simulink model "Model_IPS"  (Simulink 7.8)
settings: Solver=ode45  StartTime=0.0  StopTime=4  MaxStep=0.00001  RelTol=1e-3
values from neighbouring files (symbols this model uses):
  Imrn = 7.4    [parametriAM.m]
  Ismax = In*sqrt(2)    [parametriAM.m]
  J = 0.019    [parametriAM.m]
  Lm = 0.0493    [parametriAM.m]
  Lr = 0.05315    [parametriAM.m]
  Ls = 0.05315    [parametriAM.m]
  Ls_oc = Ls    (= 0.05315)    [parametriAM.m]
  pp = 3    [parametriAM.m]
  Rs = 0.594    [parametriAM.m]
  Rs_oc = Rs    (= 0.594)    [parametriAM.m]
  sigma = 1 - 1/((1+sigmaR)*(1+sigmaS))    (= 0.13962595434)    [parametriAM.m]
  sigma_oc = 1 - 1/((1+sigmaR_oc)*(1+sigmaS_oc))    (= 0.13962595434)    [parametriAM.m]
  Tr = Lr/Rr    (= 0.0771407837446)    [parametriAM.m]
  Usmax = Udc    [parametriAM.m]
libraries: simulink x5
settings Model: Creator=Vaje  LastModifiedBy=Mitja1  CovModelRefEnable=off
settings DataIOCC: LimitDataPoints=off  SaveFormat=StructureWithTime  SignalLoggingSaveFormat=Dataset
settings OptimizationCC: ExpressionDepthLimit=128
settings DebuggingCC: UnderspecifiedInitializationDetection=Simplified  MergeDetectMultiDrivingBlocksExec=error  SolverPrmCheckMsg=none  FrameProcessingCompatibilityMsg=error  StateNameClashWarn=none
settings HardwareCC: ProdBitPerPointer=64  ProdLargestAtomicFloat=Float  ProdIntDivRoundTo=Zero  ProdEndianess=LittleEndian  ProdHWDeviceType=Specified
settings CodeAppCC: CustomSymbolStrType=$N$R$M_T
settings GRTTargetCC: TargetFunctionLibrary=C89/C90 (ANSI)

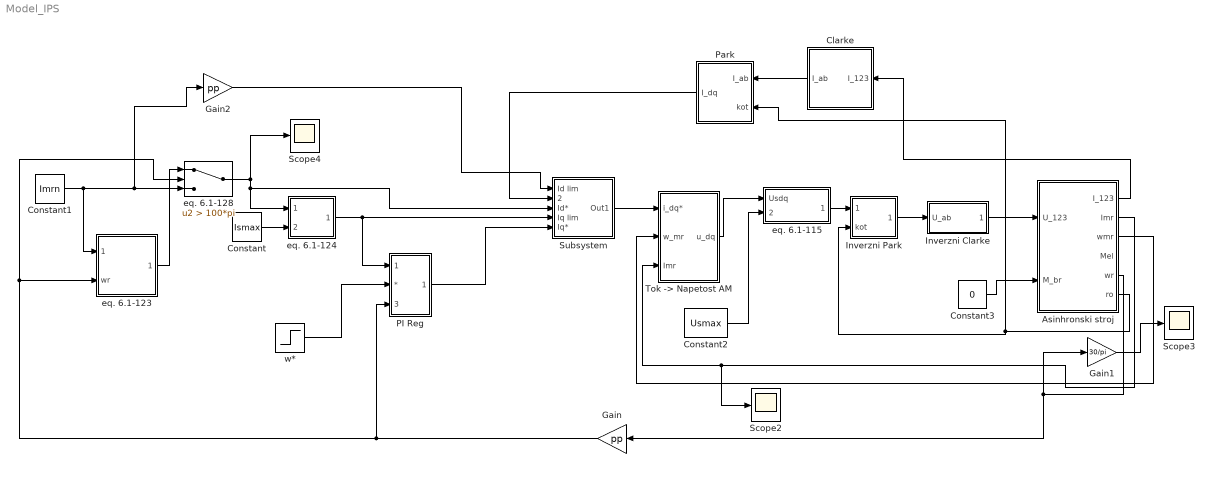
== system Model_IPS ==
  Asinhronski stroj : Subsystem  InitFcn=parametriAM
  Clarke : Subsystem
  Constant : Constant  Value=Ismax
  Constant1 : Constant  Value=Imrn
  Constant2 : Constant  Value=Usmax
  Constant3 : Constant  Value=0
  Gain : Gain  Gain=pp
  Gain1 : Gain  Gain=30/pi
  Gain2 : Gain  Gain=pp
  Inverzni Clarke : Subsystem
  Inverzni Park : Subsystem
  PI Reg : Subsystem
  Park : Subsystem
  Scope2 : Scope
      settings: TimeRange=auto  MaxDataPoints=5000  SaveToWorkspace=off  SaveName=ScopeData2  YMin=8.68295  YMax=8.68443  SampleTime=-1
  Scope3 : Scope
      settings: TimeRange=auto  MaxDataPoints=5000  SaveToWorkspace=off  SaveName=ScopeData3  YMin=-1.00000  YMax=1.00000  SampleTime=-1
  Scope4 : Scope
      settings: TimeRange=auto  MaxDataPoints=5000  SaveToWorkspace=off  SaveName=ScopeData2  YMin=0  YMax=10  SampleTime=-1
  Subsystem : Subsystem
  "Tok -> Napetost AM" : Subsystem
  eq. 6.1-115 : Subsystem
  eq. 6.1-123 : Subsystem
  eq. 6.1-124 : Subsystem
  eq. 6.1-128 : Switch  Criteria=u2 > Threshold  Threshold=100*pi
  w* : Step  Time=0.3  After=200*pi  SampleTime=0
  wires:
  Inverzni Clarke/1(U_123) -> Asinhronski stroj/1(U_123)
  Asinhronski stroj/1(I_123) -> Clarke/1(I_123)
  Asinhronski stroj/6(ro) -> Park/2(kot), Inverzni Park/2(kot)
  Inverzni Park/1(U_ab) -> Inverzni Clarke/1(U_ab)
  eq. 6.1-115/1(Usdqlim) -> Inverzni Park/1(U_dq)
  eq. 6.1-128/1 -> Subsystem/3(Id*), eq. 6.1-124/1(Isdref), Scope4/1
  eq. 6.1-123/1(Isdref) -> eq. 6.1-128/1
  Constant/1 -> eq. 6.1-124/2(Ismax)
  Constant1/1 -> eq. 6.1-123/1(Isdrated), Gain2/1, eq. 6.1-128/3
  Gain/1 -> eq. 6.1-128/2, eq. 6.1-123/2(wr), PI Reg/3(dej)
  Constant2/1 -> eq. 6.1-115/2(Usmax)
  Asinhronski stroj/5(wr) -> Gain1/1, Gain/1
  eq. 6.1-124/1(Isq lim) -> PI Reg/1(Sat), Subsystem/4(Iq lim)
  Clarke/1(I_ab) -> Park/1(I_ab)
  "Tok -> Napetost AM"/1(u_dq) -> eq. 6.1-115/1(Usdq)
  Asinhronski stroj/2(Imr) -> Scope2/1, "Tok -> Napetost AM"/3(Imr)
  Asinhronski stroj/3(wmr) -> "Tok -> Napetost AM"/2(w_mr)
  Gain1/1 -> Scope3/1
  Constant3/1 -> Asinhronski stroj/2(M_br)
  w*/1 -> PI Reg/2(*)
  Gain2/1 -> Subsystem/1(Id lim)
  Park/1(I_dq) -> Subsystem/2(Idq dej)
  PI Reg/1(Out) -> Subsystem/5(Iq*)
  Subsystem/1(Out1) -> "Tok -> Napetost AM"/1(i_dq*)

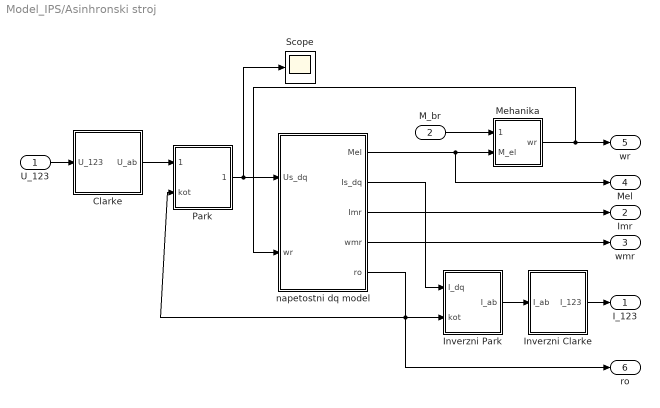
== system Model_IPS/Asinhronski stroj ==
  U_123 : Inport
  M_br : Inport  Port=2
  Clarke : Subsystem
  Inverzni Clarke : Subsystem
  Inverzni Park : Subsystem
  Mehanika : Subsystem
  Park : Subsystem
  Scope : Scope
      settings: TimeRange=auto  MaxDataPoints=5000  SaveToWorkspace=off  SaveName=ScopeData  YMin=-1.00000  YMax=1.00000  SampleTime=-1
  napetostni dq model : Subsystem
  I_123 : Outport
  Imr : Outport  Port=2
  wmr : Outport  Port=3
  Mel : Outport  Port=4
  wr : Outport  Port=5
  ro : Outport  Port=6
  wires:
  Inverzni Park/1(I_ab) -> Inverzni Clarke/1(I_ab)
  Clarke/1(U_ab) -> Park/1(U_ab)
  Mehanika/1(wr) -> napetostni dq model/2(wr), wr/1
  M_br/1 -> Mehanika/1(M_br)
  napetostni dq model/1(Mel) -> Mel/1, Mehanika/2(M_el)
  Inverzni Clarke/1(I_123) -> I_123/1
  napetostni dq model/4(wmr) -> wmr/1
  napetostni dq model/3(Imr) -> Imr/1
  U_123/1 -> Clarke/1(U_123)
  napetostni dq model/2(Is_dq) -> Inverzni Park/1(I_dq)
  napetostni dq model/5(ro) -> ro/1, Park/2(kot), Inverzni Park/2(kot)
  Park/1(U_dq) -> Scope/1, napetostni dq model/1(Us_dq)

== system Model_IPS/Clarke ==
  I_123 : Inport
  ABC_ab1 : Subsystem
  Demux : Demux  Outputs=3
  Mux : Mux  Inputs=2
  I_ab : Outport
  wires:
  Mux/1 -> I_ab/1
  ABC_ab1/2(beta) -> Mux/2
  ABC_ab1/1(alfa) -> Mux/1
  Demux/3 -> ABC_ab1/3(C)
  Demux/2 -> ABC_ab1/2(B)
  Demux/1 -> ABC_ab1/1(A)
  I_123/1 -> Demux/1

== system Model_IPS/Inverzni Clarke ==
  U_ab : Inport
  Demux : Demux  Outputs=2
  Mux : Mux  Inputs=3
  ab_ABC : Subsystem
  U_123 : Outport
  wires:
  ab_ABC/3(C) -> Mux/3
  ab_ABC/2(B) -> Mux/2
  ab_ABC/1(A) -> Mux/1
  Demux/2 -> ab_ABC/2(beta)
  Demux/1 -> ab_ABC/1(alfa)
  U_ab/1 -> Demux/1
  Mux/1 -> U_123/1

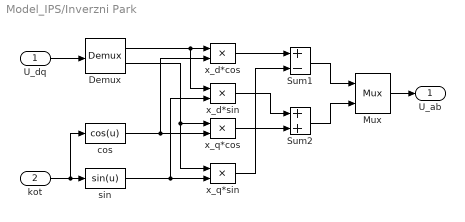
== system Model_IPS/Inverzni Park ==
  U_dq : Inport
  kot : Inport  Port=2
  Demux : Demux  Outputs=2
  Mux : Mux  Inputs=2
  "Sum1 " : Sum  Inputs=+-  SaturateOnIntegerOverflow=on  InputSameDT=on  OutDataTypeStr=Inherit: Same as first input
  Sum2 : Sum  SaturateOnIntegerOverflow=on  InputSameDT=on  OutDataTypeStr=Inherit: Same as first input
  cos : Fcn  Expr=cos(u)
  sin : Fcn  Expr=sin(u)
  x_d*cos : Product  SaturateOnIntegerOverflow=on  RndMeth=Zero  InputSameDT=on  OutDataTypeStr=Inherit: Same as first input
  x_d*sin : Product  SaturateOnIntegerOverflow=on  RndMeth=Zero  InputSameDT=on  OutDataTypeStr=Inherit: Same as first input
  x_q*cos : Product  SaturateOnIntegerOverflow=on  RndMeth=Zero  InputSameDT=on  OutDataTypeStr=Inherit: Same as first input
  "x_q*sin " : Product  SaturateOnIntegerOverflow=on  RndMeth=Zero  InputSameDT=on  OutDataTypeStr=Inherit: Same as first input
  U_ab : Outport
  wires:
  Mux/1 -> U_ab/1
  U_dq/1 -> Demux/1
  Demux/1 -> x_d*sin/1, x_d*cos/1
  Demux/2 -> "x_q*sin "/1, x_q*cos/1
  cos/1 -> x_q*cos/2, x_d*cos/2
  sin/1 -> "x_q*sin "/2, x_d*sin/2
  x_d*cos/1 -> "Sum1 "/1
  "x_q*sin "/1 -> "Sum1 "/2
  x_q*cos/1 -> Sum2/2
  x_d*sin/1 -> Sum2/1
  "Sum1 "/1 -> Mux/1
  Sum2/1 -> Mux/2
  kot/1 -> cos/1, sin/1

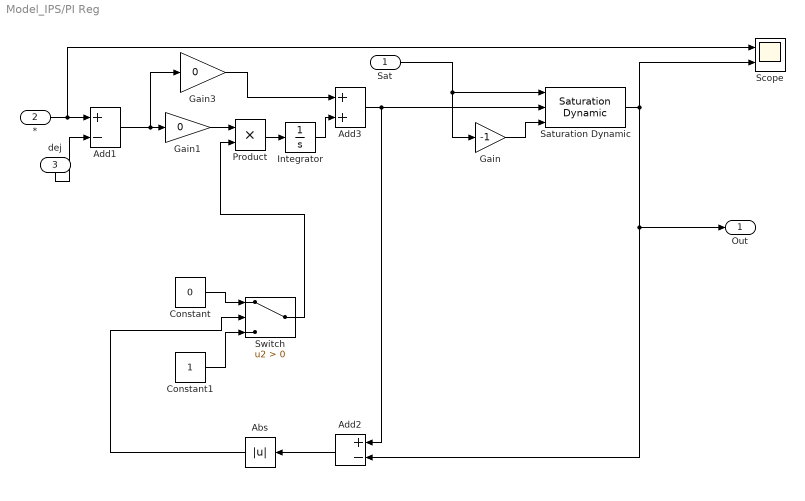
== system Model_IPS/PI Reg ==
  Sat : Inport
  * : Inport  Port=2
  dej : Inport  Port=3
  Abs : Abs
  Add1 : Sum  Inputs=+-
  Add2 : Sum  Inputs=+-
  Add3 : Sum
  Constant : Constant  Value=0
  Constant1 : Constant
  Gain : Gain  Gain=-1
  Gain1 : Gain  Gain=0
  Gain3 : Gain  Gain=0
  Integrator : Integrator
  Product : Product
  Saturation Dynamic : simulink/Discontinuities/Saturation Dynamic  OutMin=[]  OutMax=[]  OutDataTypeStr=Inherit: Same as second input  OutDataType=fixdt(1, 16)  OutScaling=2^-10  DoSatur=off
  Scope : Scope  NumInputPorts=2
      settings: TimeRange=auto  MaxDataPoints=5000  SaveToWorkspace=off  SaveName=ScopeData7  YMin=-2.0166~-5  YMax=2.47044~5  SampleTime=-1
  Switch : Switch  Criteria=u2 > Threshold  ZeroCross=off
  Out : Outport
  wires:
  Product/1 -> Integrator/1
  dej/1 -> Add1/2
  Constant1/1 -> Switch/3
  Gain3/1 -> Add3/1
  */1 -> Scope/1, Add1/1
  Saturation Dynamic/1 -> Add2/2, Out/1, Scope/2
  Add2/1 -> Abs/1
  Integrator/1 -> Add3/2
  Gain1/1 -> Product/1
  Add1/1 -> Gain1/1, Gain3/1
  Add3/1 -> Add2/1, Saturation Dynamic/2
  Switch/1 -> Product/2
  Constant/1 -> Switch/1
  Abs/1 -> Switch/2
  Sat/1 -> Saturation Dynamic/1, Gain/1
  Gain/1 -> Saturation Dynamic/3

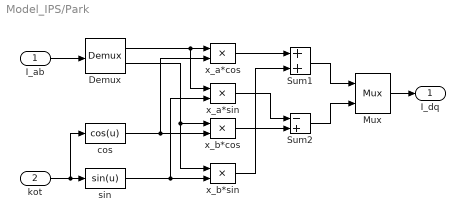
== system Model_IPS/Park ==
  I_ab : Inport
  kot : Inport  Port=2
  Demux : Demux  Outputs=2
  Mux : Mux  Inputs=2
  "Sum1 " : Sum  SaturateOnIntegerOverflow=on  InputSameDT=on  OutDataTypeStr=Inherit: Same as first input
  Sum2 : Sum  Inputs=-+  SaturateOnIntegerOverflow=on  InputSameDT=on  OutDataTypeStr=Inherit: Same as first input
  cos : Fcn  Expr=cos(u)
  sin : Fcn  Expr=sin(u)
  x_a*cos : Product  SaturateOnIntegerOverflow=on  RndMeth=Zero  InputSameDT=on  OutDataTypeStr=Inherit: Same as first input
  x_a*sin : Product  SaturateOnIntegerOverflow=on  RndMeth=Zero  InputSameDT=on  OutDataTypeStr=Inherit: Same as first input
  x_b*cos : Product  SaturateOnIntegerOverflow=on  RndMeth=Zero  InputSameDT=on  OutDataTypeStr=Inherit: Same as first input
  "x_b*sin " : Product  SaturateOnIntegerOverflow=on  RndMeth=Zero  InputSameDT=on  OutDataTypeStr=Inherit: Same as first input
  I_dq : Outport
  wires:
  Mux/1 -> I_dq/1
  I_ab/1 -> Demux/1
  Demux/1 -> x_a*sin/1, x_a*cos/1
  Demux/2 -> "x_b*sin "/1, x_b*cos/1
  cos/1 -> x_b*cos/2, x_a*cos/2
  sin/1 -> "x_b*sin "/2, x_a*sin/2
  x_a*cos/1 -> "Sum1 "/1
  "x_b*sin "/1 -> "Sum1 "/2
  x_b*cos/1 -> Sum2/2
  x_a*sin/1 -> Sum2/1
  "Sum1 "/1 -> Mux/1
  Sum2/1 -> Mux/2
  kot/1 -> cos/1, sin/1

== system Model_IPS/Subsystem ==
  Id lim : Inport
  Idq dej : Inport  Port=2
  Id* : Inport  Port=3
  Iq lim : Inport  Port=4
  Iq* : Inport  Port=5
  Demux : Demux  Outputs=2
  Mux : Mux  Inputs=2
  PI Id : Subsystem
  PI Iq : Subsystem
  Scope6 : Scope  NumInputPorts=2
      settings: TimeRange=auto  MaxDataPoints=5000  SaveToWorkspace=off  SaveName=ScopeData4  YMin=-6.22165~-5  YMax=55.99486~5  SampleTime=-1
  Out1 : Outport
  wires:
  Id*/1 -> Scope6/1, PI Id/2(*)
  Iq lim/1 -> PI Iq/1(Sat)
  PI Id/1(Out) -> Mux/1, Scope6/2
  Demux/2 -> PI Iq/3(dej)
  Iq*/1 -> PI Iq/2(*)
  Id lim/1 -> PI Id/1(Sat)
  Demux/1 -> PI Id/3(dej)
  PI Iq/1(Out) -> Mux/2
  Mux/1 -> Out1/1
  Idq dej/1 -> Demux/1

== system Model_IPS/Tok -> Napetost AM ==
  i_dq* : Inport
  w_mr : Inport  Port=2
  Imr : Inport  Port=3
  Mux : Mux  Inputs=2
  eq 5.146 : Subsystem
  eq 5.147 : Subsystem
  u_dq : Outport
  wires:
  i_dq*/1 -> eq 5.147/1(I_dq), eq 5.146/1(I_dq)
  Mux/1 -> u_dq/1
  w_mr/1 -> eq 5.147/2(w_mr), eq 5.146/2(w_mr)
  Imr/1 -> eq 5.146/3(Imr), eq 5.147/3(Imr)
  eq 5.147/1(u_q) -> Mux/2
  eq 5.146/1(u_d) -> Mux/1

== system Model_IPS/eq. 6.1-115 ==
  Usdq : Inport
  Usmax : Inport  Port=2
  Demux : Demux  Outputs=2
  Mux1 : Mux  Inputs=2
  eq. 6.1-120 : Subsystem
  eq. 6.1-120a : Subsystem
  Usdqlim : Outport
  wires:
  Mux1/1 -> Usdqlim/1
  eq. 6.1-120a/1(Usqlim) -> Mux1/2
  eq. 6.1-120/1(Usdlim) -> Mux1/1
  Usdq/1 -> Demux/1
  Demux/1 -> eq. 6.1-120a/1(Usd), eq. 6.1-120/2(Usd)
  Demux/2 -> eq. 6.1-120a/2(Usq), eq. 6.1-120/1(Usq)
  Usmax/1 -> eq. 6.1-120/3(Usmax), eq. 6.1-120a/3(Usmax)

== system Model_IPS/eq. 6.1-123 ==
  Isdrated : Inport
  wr : Inport  Port=2
  Divide : Product  Inputs=*/
  Gain : Gain  Gain=100*pi
  Isdref : Outport
  wires:
  wr/1 -> Divide/2
  Isdrated/1 -> Divide/1
  Gain/1 -> Isdref/1
  Divide/1 -> Gain/1

== system Model_IPS/eq. 6.1-124 ==
  Isdref : Inport
  Ismax : Inport  Port=2
  Add : Sum  Inputs=+-
  Product : Product
  Product1 : Product
  Sqrt : Sqrt  SaturateOnIntegerOverflow=on
  Isq lim : Outport
  wires:
  Ismax/1 -> Product/2, Product/1
  Product1/1 -> Add/2
  Product/1 -> Add/1
  Add/1 -> Sqrt/1
  Isdref/1 -> Product1/2, Product1/1
  Sqrt/1 -> Isq lim/1

== system Model_IPS/Asinhronski stroj/Clarke ==
  U_123 : Inport
  ABC_ab1 : Subsystem
  Demux : Demux  Outputs=3
  Mux : Mux  Inputs=2
  U_ab : Outport
  wires:
  Mux/1 -> U_ab/1
  ABC_ab1/2(beta) -> Mux/2
  ABC_ab1/1(alfa) -> Mux/1
  Demux/3 -> ABC_ab1/3(C)
  Demux/2 -> ABC_ab1/2(B)
  Demux/1 -> ABC_ab1/1(A)
  U_123/1 -> Demux/1

== system Model_IPS/Asinhronski stroj/Inverzni Clarke ==
  I_ab : Inport
  Demux : Demux  Outputs=2
  Mux : Mux  Inputs=3
  ab_ABC : Subsystem
  I_123 : Outport
  wires:
  ab_ABC/3(C) -> Mux/3
  ab_ABC/2(B) -> Mux/2
  ab_ABC/1(A) -> Mux/1
  Demux/2 -> ab_ABC/2(beta)
  Demux/1 -> ab_ABC/1(alfa)
  I_ab/1 -> Demux/1
  Mux/1 -> I_123/1

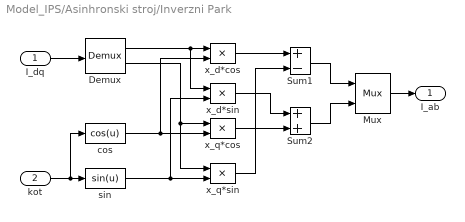
== system Model_IPS/Asinhronski stroj/Inverzni Park ==
  I_dq : Inport
  kot : Inport  Port=2
  Demux : Demux  Outputs=2
  Mux : Mux  Inputs=2
  "Sum1 " : Sum  Inputs=+-  SaturateOnIntegerOverflow=on  InputSameDT=on  OutDataTypeStr=Inherit: Same as first input
  Sum2 : Sum  SaturateOnIntegerOverflow=on  InputSameDT=on  OutDataTypeStr=Inherit: Same as first input
  cos : Fcn  Expr=cos(u)
  sin : Fcn  Expr=sin(u)
  x_d*cos : Product  SaturateOnIntegerOverflow=on  RndMeth=Zero  InputSameDT=on  OutDataTypeStr=Inherit: Same as first input
  x_d*sin : Product  SaturateOnIntegerOverflow=on  RndMeth=Zero  InputSameDT=on  OutDataTypeStr=Inherit: Same as first input
  x_q*cos : Product  SaturateOnIntegerOverflow=on  RndMeth=Zero  InputSameDT=on  OutDataTypeStr=Inherit: Same as first input
  "x_q*sin " : Product  SaturateOnIntegerOverflow=on  RndMeth=Zero  InputSameDT=on  OutDataTypeStr=Inherit: Same as first input
  I_ab : Outport
  wires:
  Mux/1 -> I_ab/1
  I_dq/1 -> Demux/1
  Demux/1 -> x_d*sin/1, x_d*cos/1
  Demux/2 -> "x_q*sin "/1, x_q*cos/1
  cos/1 -> x_q*cos/2, x_d*cos/2
  sin/1 -> "x_q*sin "/2, x_d*sin/2
  x_d*cos/1 -> "Sum1 "/1
  "x_q*sin "/1 -> "Sum1 "/2
  x_q*cos/1 -> Sum2/2
  x_d*sin/1 -> Sum2/1
  "Sum1 "/1 -> Mux/1
  Sum2/1 -> Mux/2
  kot/1 -> cos/1, sin/1

== system Model_IPS/Asinhronski stroj/Mehanika ==
  M_br : Inport
  M_el : Inport  Port=2
  Sum : Sum  Inputs=+-
  eq 2.19 : Subsystem
  wr : Outport
  wires:
  M_br/1 -> Sum/2
  Sum/1 -> eq 2.19/1(M)
  M_el/1 -> Sum/1
  eq 2.19/1(wr) -> wr/1

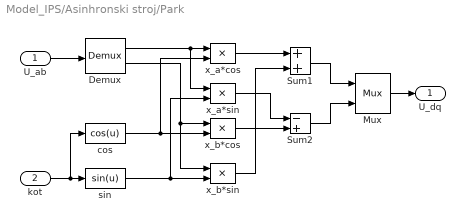
== system Model_IPS/Asinhronski stroj/Park ==
  U_ab : Inport
  kot : Inport  Port=2
  Demux : Demux  Outputs=2
  Mux : Mux  Inputs=2
  "Sum1 " : Sum  SaturateOnIntegerOverflow=on  InputSameDT=on  OutDataTypeStr=Inherit: Same as first input
  Sum2 : Sum  Inputs=-+  SaturateOnIntegerOverflow=on  InputSameDT=on  OutDataTypeStr=Inherit: Same as first input
  cos : Fcn  Expr=cos(u)
  sin : Fcn  Expr=sin(u)
  x_a*cos : Product  SaturateOnIntegerOverflow=on  RndMeth=Zero  InputSameDT=on  OutDataTypeStr=Inherit: Same as first input
  x_a*sin : Product  SaturateOnIntegerOverflow=on  RndMeth=Zero  InputSameDT=on  OutDataTypeStr=Inherit: Same as first input
  x_b*cos : Product  SaturateOnIntegerOverflow=on  RndMeth=Zero  InputSameDT=on  OutDataTypeStr=Inherit: Same as first input
  "x_b*sin " : Product  SaturateOnIntegerOverflow=on  RndMeth=Zero  InputSameDT=on  OutDataTypeStr=Inherit: Same as first input
  U_dq : Outport
  wires:
  Mux/1 -> U_dq/1
  U_ab/1 -> Demux/1
  Demux/1 -> x_a*sin/1, x_a*cos/1
  Demux/2 -> "x_b*sin "/1, x_b*cos/1
  cos/1 -> x_b*cos/2, x_a*cos/2
  sin/1 -> "x_b*sin "/2, x_a*sin/2
  x_a*cos/1 -> "Sum1 "/1
  "x_b*sin "/1 -> "Sum1 "/2
  x_b*cos/1 -> Sum2/2
  x_a*sin/1 -> Sum2/1
  "Sum1 "/1 -> Mux/1
  Sum2/1 -> Mux/2
  kot/1 -> cos/1, sin/1

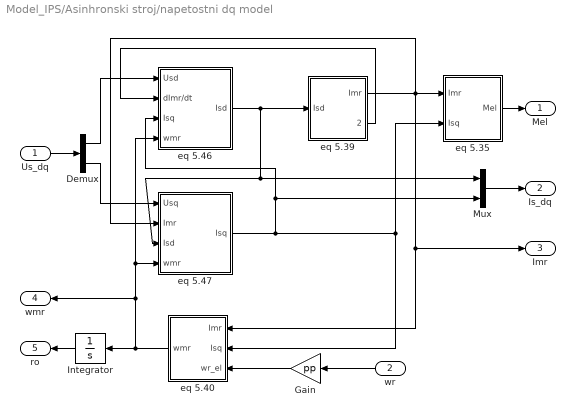
== system Model_IPS/Asinhronski stroj/napetostni dq model ==
  Us_dq : Inport
  wr : Inport  Port=2
  Demux : Demux  Outputs=2
  Gain : Gain  Gain=pp
  Integrator : Integrator
  Mux : Mux  Inputs=2
  eq 5.35 : Subsystem
  eq 5.39 : Subsystem
  eq 5.40 : Subsystem
  eq 5.46 : Subsystem
  eq 5.47 : Subsystem
  Mel : Outport
  Is_dq : Outport  Port=2
  Imr : Outport  Port=3
  wmr : Outport  Port=4
  ro : Outport  Port=5
  wires:
  Gain/1 -> eq 5.40/3(wr_el)
  Mux/1 -> Is_dq/1
  Demux/2 -> eq 5.47/1(Usq)
  Demux/1 -> eq 5.46/1(Usd)
  Us_dq/1 -> Demux/1
  wr/1 -> Gain/1
  Integrator/1 -> ro/1
  eq 5.35/1(Mel) -> Mel/1
  eq 5.40/1(wmr) -> Integrator/1, wmr/1, eq 5.46/4(wmr), eq 5.47/4(wmr)
  eq 5.47/1(Isq) -> Mux/2, eq 5.46/3(Isq), eq 5.40/2(Isq), eq 5.35/2(Isq)
  eq 5.39/1(Imr) -> eq 5.47/2(Imr), Imr/1, eq 5.40/1(Imr), eq 5.35/1(Imr)
  eq 5.39/2(dImr/dt) -> eq 5.46/2(dImr/dt)
  eq 5.46/1(Isd) -> Mux/1, eq 5.47/3(Isd), eq 5.39/1(Isd)

== system Model_IPS/Clarke/ABC_ab1 ==
  A : Inport
  B : Inport  Port=2
  C : Inport  Port=3
  Gain1 : Gain  Gain=2
  Gain2 : Gain
  Gain24 : Gain  Gain=sqrt(3)/3
  Sum11 : Sum
  Terminator : Terminator
  alfa : Outport
  beta : Outport  Port=2
  wires:
  C/1 -> Terminator/1
  Gain1/1 -> Sum11/2
  B/1 -> Gain1/1
  Gain24/1 -> beta/1
  Gain2/1 -> alfa/1
  Sum11/1 -> Gain24/1
  A/1 -> Sum11/1, Gain2/1

== system Model_IPS/Inverzni Clarke/ab_ABC ==
  alfa : Inport
  beta : Inport  Port=2
  Gain1 : Gain
  Gain2 : Gain  Gain=-0.5
  Gain25 : Gain  Gain=sqrt(3)/2
  Gain3 : Gain  Gain=sqrt(3)/2
  Gain4 : Gain  Gain=0.5
  Sum10 : Sum
  Sum11 : Sum  Inputs=--
  A : Outport
  B : Outport  Port=2
  C : Outport  Port=3
  wires:
  Gain3/1 -> Sum11/2
  beta/1 -> Gain25/1, Gain3/1
  Gain4/1 -> Sum11/1
  Gain25/1 -> Sum10/2
  Gain2/1 -> Sum10/1
  alfa/1 -> Gain1/1, Gain2/1, Gain4/1
  Gain1/1 -> A/1
  Sum10/1 -> B/1
  Sum11/1 -> C/1

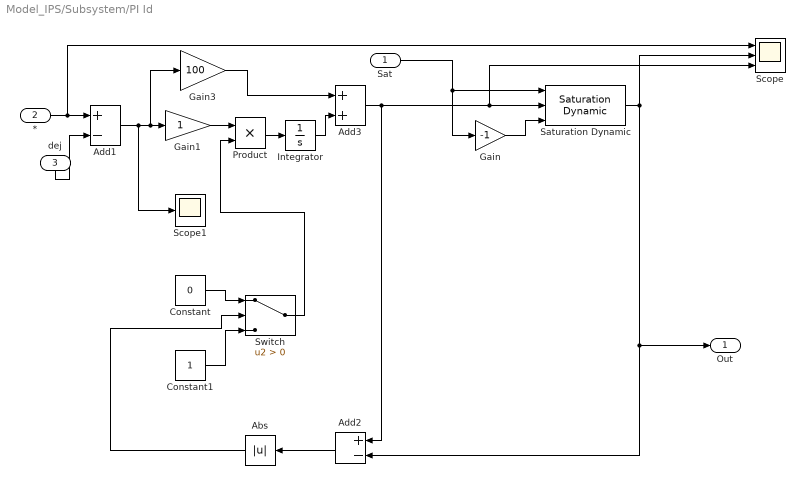
== system Model_IPS/Subsystem/PI Id ==
  Sat : Inport
  * : Inport  Port=2
  dej : Inport  Port=3
  Abs : Abs
  Add1 : Sum  Inputs=+-
  Add2 : Sum  Inputs=+-
  Add3 : Sum
  Constant : Constant  Value=0
  Constant1 : Constant
  Gain : Gain  Gain=-1
  Gain1 : Gain
  Gain3 : Gain  Gain=100
  Integrator : Integrator
  Product : Product
  Saturation Dynamic : simulink/Discontinuities/Saturation Dynamic  OutMin=[]  OutMax=[]  OutDataTypeStr=Inherit: Same as second input  OutDataType=fixdt(1, 16)  OutScaling=2^-10  DoSatur=off
  Scope : Scope  NumInputPorts=3
      settings: TimeRange=auto  MaxDataPoints=5000  SaveToWorkspace=off  SaveName=ScopeData7  YMin=6.04784~-5~-5  YMax=9.06135~5~5  SampleTime=-1
  Scope1 : Scope
      settings: TimeRange=auto  MaxDataPoints=5000  SaveToWorkspace=off  YMin=-0.02022  YMax=0.13918  SampleTime=-1
  Switch : Switch  Criteria=u2 > Threshold  ZeroCross=off
  Out : Outport
  wires:
  Gain/1 -> Saturation Dynamic/3
  Sat/1 -> Gain/1, Saturation Dynamic/1
  Abs/1 -> Switch/2
  Constant/1 -> Switch/1
  Switch/1 -> Product/2
  Add3/1 -> Scope/3, Saturation Dynamic/2, Add2/1
  Add1/1 -> Scope1/1, Gain3/1, Gain1/1
  Gain1/1 -> Product/1
  Integrator/1 -> Add3/2
  Add2/1 -> Abs/1
  Saturation Dynamic/1 -> Scope/2, Out/1, Add2/2
  */1 -> Add1/1, Scope/1
  Gain3/1 -> Add3/1
  Constant1/1 -> Switch/3
  dej/1 -> Add1/2
  Product/1 -> Integrator/1

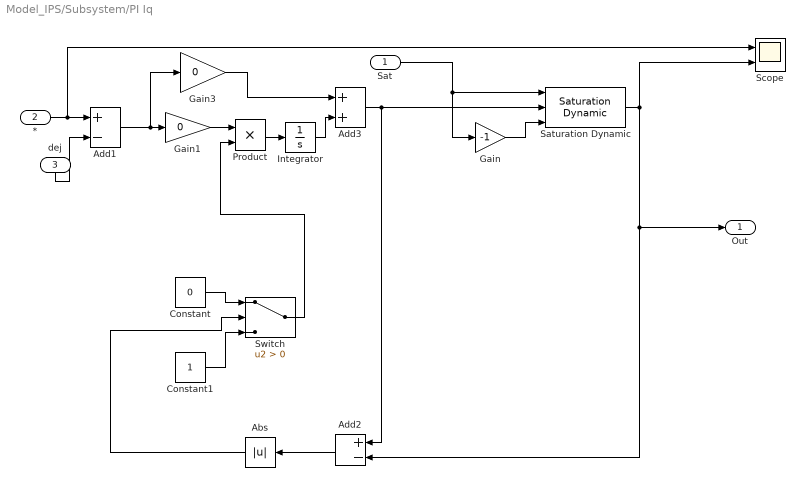
== system Model_IPS/Subsystem/PI Iq ==
  Sat : Inport
  * : Inport  Port=2
  dej : Inport  Port=3
  Abs : Abs
  Add1 : Sum  Inputs=+-
  Add2 : Sum  Inputs=+-
  Add3 : Sum
  Constant : Constant  Value=0
  Constant1 : Constant
  Gain : Gain  Gain=-1
  Gain1 : Gain  Gain=0
  Gain3 : Gain  Gain=0
  Integrator : Integrator
  Product : Product
  Saturation Dynamic : simulink/Discontinuities/Saturation Dynamic  OutMin=[]  OutMax=[]  OutDataTypeStr=Inherit: Same as second input  OutDataType=fixdt(1, 16)  OutScaling=2^-10  DoSatur=off
  Scope : Scope  NumInputPorts=2
      settings: TimeRange=auto  MaxDataPoints=5000  SaveToWorkspace=off  SaveName=ScopeData7  YMin=-2.0166~-5  YMax=2.47044~5  SampleTime=-1
  Switch : Switch  Criteria=u2 > Threshold  ZeroCross=off
  Out : Outport
  wires:
  Product/1 -> Integrator/1
  dej/1 -> Add1/2
  Constant1/1 -> Switch/3
  Gain3/1 -> Add3/1
  */1 -> Scope/1, Add1/1
  Saturation Dynamic/1 -> Add2/2, Out/1, Scope/2
  Add2/1 -> Abs/1
  Integrator/1 -> Add3/2
  Gain1/1 -> Product/1
  Add1/1 -> Gain1/1, Gain3/1
  Add3/1 -> Add2/1, Saturation Dynamic/2
  Switch/1 -> Product/2
  Constant/1 -> Switch/1
  Abs/1 -> Switch/2
  Sat/1 -> Saturation Dynamic/1, Gain/1
  Gain/1 -> Saturation Dynamic/3

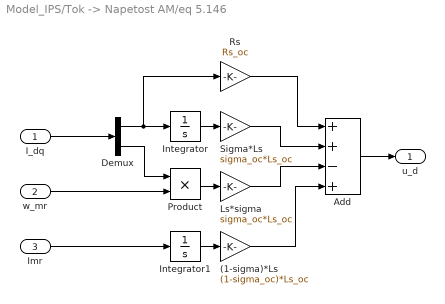
== system Model_IPS/Tok -> Napetost AM/eq 5.146 ==
  I_dq : Inport
  w_mr : Inport  Port=2
  Imr : Inport  Port=3
  (1-sigma)*Ls : Gain  Gain=(1-sigma_oc)*Ls_oc
  Add : Sum  Inputs=++-+
  Demux : Demux  Outputs=2
  Integrator : Integrator
  Integrator1 : Integrator
  Ls*sigma : Gain  Gain=sigma_oc*Ls_oc
  Product : Product
  Rs : Gain  Gain=Rs_oc
  Sigma*Ls : Gain  Gain=sigma_oc*Ls_oc
  u_d : Outport
  wires:
  w_mr/1 -> Product/2
  Product/1 -> Ls*sigma/1
  Demux/2 -> Product/1
  (1-sigma)*Ls/1 -> Add/4
  Integrator/1 -> Sigma*Ls/1
  Rs/1 -> Add/1
  Sigma*Ls/1 -> Add/2
  Integrator1/1 -> (1-sigma)*Ls/1
  Demux/1 -> Integrator/1, Rs/1
  Ls*sigma/1 -> Add/3
  Add/1 -> u_d/1
  I_dq/1 -> Demux/1
  Imr/1 -> Integrator1/1

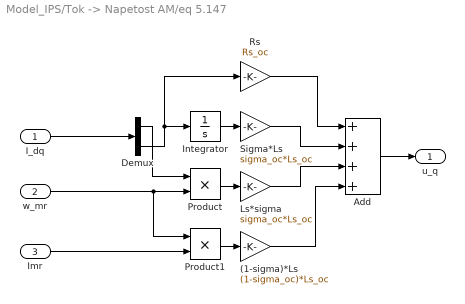
== system Model_IPS/Tok -> Napetost AM/eq 5.147 ==
  I_dq : Inport
  w_mr : Inport  Port=2
  Imr : Inport  Port=3
  (1-sigma)*Ls : Gain  Gain=(1-sigma_oc)*Ls_oc
  Add : Sum  Inputs=++++
  Demux : Demux  Outputs=2
  Integrator : Integrator
  Ls*sigma : Gain  Gain=sigma_oc*Ls_oc
  Product : Product
  Product1 : Product
  Rs : Gain  Gain=Rs_oc
  Sigma*Ls : Gain  Gain=sigma_oc*Ls_oc
  u_q : Outport
  wires:
  w_mr/1 -> Product1/1, Product/2
  Product/1 -> Ls*sigma/1
  (1-sigma)*Ls/1 -> Add/4
  Integrator/1 -> Sigma*Ls/1
  Rs/1 -> Add/1
  Sigma*Ls/1 -> Add/2
  Ls*sigma/1 -> Add/3
  Add/1 -> u_q/1
  I_dq/1 -> Demux/1
  Demux/2 -> Integrator/1, Rs/1
  Demux/1 -> Product/1
  Product1/1 -> (1-sigma)*Ls/1
  Imr/1 -> Product1/2

== system Model_IPS/eq. 6.1-115/eq. 6.1-120 ==
  Usq : Inport
  Usd : Inport  Port=2
  Usmax : Inport  Port=3
  Add : Sum
  Gain : Gain  Gain=-1
  Product : Product
  Product1 : Product
  Saturation Dynamic : simulink/Discontinuities/Saturation Dynamic  OutMin=[]  OutMax=[]  OutDataTypeStr=Inherit: Same as second input  OutDataType=fixdt(1, 16)  OutScaling=2^-10  DoSatur=off
  Sqrt : Sqrt  SaturateOnIntegerOverflow=on
  Usdlim : Outport
  wires:
  Usd/1 -> Saturation Dynamic/2
  Saturation Dynamic/1 -> Usdlim/1
  Usq/1 -> Product1/1, Product1/2
  Gain/1 -> Saturation Dynamic/3
  Add/1 -> Sqrt/1
  Product/1 -> Add/1
  Sqrt/1 -> Gain/1, Saturation Dynamic/1
  Product1/1 -> Add/2
  Usmax/1 -> Product/1, Product/2

== system Model_IPS/eq. 6.1-115/eq. 6.1-120a ==
  Usd : Inport
  Usq : Inport  Port=2
  Usmax : Inport  Port=3
  Add : Sum
  Gain : Gain  Gain=-1
  Product : Product
  Product1 : Product
  Saturation Dynamic : simulink/Discontinuities/Saturation Dynamic  OutMin=[]  OutMax=[]  OutDataTypeStr=Inherit: Same as second input  OutDataType=fixdt(1, 16)  OutScaling=2^-10  DoSatur=off
  Sqrt : Sqrt  SaturateOnIntegerOverflow=on
  Usqlim : Outport
  wires:
  Usmax/1 -> Product/2, Product/1
  Product1/1 -> Add/2
  Sqrt/1 -> Saturation Dynamic/1, Gain/1
  Product/1 -> Add/1
  Add/1 -> Sqrt/1
  Gain/1 -> Saturation Dynamic/3
  Usd/1 -> Product1/2, Product1/1
  Saturation Dynamic/1 -> Usqlim/1
  Usq/1 -> Saturation Dynamic/2

== system Model_IPS/Asinhronski stroj/Clarke/ABC_ab1 ==
  A : Inport
  B : Inport  Port=2
  C : Inport  Port=3
  Gain1 : Gain  Gain=2
  Gain2 : Gain
  Gain24 : Gain  Gain=sqrt(3)/3
  Sum11 : Sum
  Terminator : Terminator
  alfa : Outport
  beta : Outport  Port=2
  wires:
  C/1 -> Terminator/1
  Gain1/1 -> Sum11/2
  B/1 -> Gain1/1
  Gain24/1 -> beta/1
  Gain2/1 -> alfa/1
  Sum11/1 -> Gain24/1
  A/1 -> Sum11/1, Gain2/1

== system Model_IPS/Asinhronski stroj/Inverzni Clarke/ab_ABC ==
  alfa : Inport
  beta : Inport  Port=2
  Gain1 : Gain
  Gain2 : Gain  Gain=-0.5
  Gain25 : Gain  Gain=sqrt(3)/2
  Gain3 : Gain  Gain=sqrt(3)/2
  Gain4 : Gain  Gain=0.5
  Sum10 : Sum
  Sum11 : Sum  Inputs=--
  A : Outport
  B : Outport  Port=2
  C : Outport  Port=3
  wires:
  Gain3/1 -> Sum11/2
  beta/1 -> Gain25/1, Gain3/1
  Gain4/1 -> Sum11/1
  Gain25/1 -> Sum10/2
  Gain2/1 -> Sum10/1
  alfa/1 -> Gain1/1, Gain2/1, Gain4/1
  Gain1/1 -> A/1
  Sum10/1 -> B/1
  Sum11/1 -> C/1

== system Model_IPS/Asinhronski stroj/Mehanika/eq 2.19 ==
  M : Inport
  Gain1 : Gain  Gain=1/J
  Integrator : Integrator
  wr : Outport
  wires:
  Integrator/1 -> wr/1
  M/1 -> Gain1/1
  Gain1/1 -> Integrator/1

== system Model_IPS/Asinhronski stroj/napetostni dq model/eq 5.35 ==
  Imr : Inport
  Isq : Inport  Port=2
  Gain : Gain  Gain=3*pp/2
  Gain2 : Gain  Gain=Lm*Lm/Lr
  Product : Product  RndMeth=Zero
  Mel : Outport
  wires:
  Gain/1 -> Gain2/1
  Gain2/1 -> Mel/1
  Product/1 -> Gain/1
  Isq/1 -> Product/2
  Imr/1 -> Product/1

== system Model_IPS/Asinhronski stroj/napetostni dq model/eq 5.39 ==
  Isd : Inport
  Gain : Gain  Gain=1/Tr
  Integrator : Integrator  InitialCondition=1e-3
  Sum : Sum  Inputs=|+-
  Imr : Outport
  dImr/dt : Outport  Port=2
  wires:
  Gain/1 -> dImr/dt/1, Integrator/1
  Sum/1 -> Gain/1
  Integrator/1 -> Sum/2, Imr/1
  Isd/1 -> Sum/1

== system Model_IPS/Asinhronski stroj/napetostni dq model/eq 5.40 ==
  Imr : Inport
  Isq : Inport  Port=2
  wr_el : Inport  Port=3
  Divide : Product  Inputs=*/
  Gain2 : Gain  Gain=Tr
  Saturation : Saturate  UpperLimit=2*pi*50  LowerLimit=-2*pi*50
  Sum : Sum  Inputs=|++
  wmr : Outport
  wires:
  Saturation/1 -> Sum/1
  Sum/1 -> wmr/1
  wr_el/1 -> Sum/2
  Divide/1 -> Saturation/1  "ws"
  Gain2/1 -> Divide/2
  Imr/1 -> Gain2/1
  Isq/1 -> Divide/1

== system Model_IPS/Asinhronski stroj/napetostni dq model/eq 5.46 ==
  Usd : Inport
  dImr/dt : Inport  Port=2
  Isq : Inport  Port=3
  wmr : Inport  Port=4
  Gain : Gain  Gain=1/(sigma*Ls)
  Gain1 : Gain  Gain=Rs
  Gain2 : Gain  Gain=(1-sigma)*Ls
  Gain3 : Gain  Gain=sigma*Ls
  Integrator : Integrator
  Product : Product  RndMeth=Zero
  Sum : Sum  Inputs=+--+
  Isd : Outport
  wires:
  Gain3/1 -> Sum/4
  Product/1 -> Gain3/1
  Isq/1 -> Product/1
  wmr/1 -> Product/2
  Gain2/1 -> Sum/3
  dImr/dt/1 -> Gain2/1
  Gain1/1 -> Sum/2
  Usd/1 -> Sum/1
  Sum/1 -> Gain/1
  Gain/1 -> Integrator/1
  Integrator/1 -> Gain1/1, Isd/1

== system Model_IPS/Asinhronski stroj/napetostni dq model/eq 5.47 ==
  Usq : Inport
  Imr : Inport  Port=2
  Isd : Inport  Port=3
  wmr : Inport  Port=4
  Gain : Gain  Gain=1/(sigma*Ls)
  Gain1 : Gain  Gain=Rs
  Gain2 : Gain  Gain=(1-sigma)*Ls
  Gain3 : Gain  Gain=sigma*Ls
  Integrator : Integrator
  Product : Product  RndMeth=Zero
  Product1 : Product  RndMeth=Zero
  Sum : Sum  Inputs=+---
  Isq : Outport
  wires:
  Gain3/1 -> Sum/4
  Product1/1 -> Gain3/1
  Isd/1 -> Product1/2
  Gain2/1 -> Sum/3
  Product/1 -> Gain2/1
  wmr/1 -> Product1/1, Product/2
  Imr/1 -> Product/1
  Gain1/1 -> Sum/2
  Usq/1 -> Sum/1
  Sum/1 -> Gain/1
  Gain/1 -> Integrator/1
  Integrator/1 -> Gain1/1, Isq/1
